simulink model "gsm_gprs_sim900_demo"  (Simulink 7.3)
settings: Solver=FixedStepDiscrete  SolverMode=SingleTasking  StartTime=0.0  StopTime=10.0  RelTol=1e-3
PreLoadFcn:
  | waijung.modelPreload; % Required for working with Waijung Blockset. Do not remove.
undefined symbols (not defined in the file): HSEOSC, Link, LQFP176, ST, STM32F417IG
libraries: waijung_atcmd_gsmgprs_lib x4, waijung_string_manipulate x4, simulink x3, waijung_systimer_lib x2, stm32f4_device_config_lib x1, stm32f4_io_lib x1
CloseFcn:
  | waijung.modelClose; % Required for working with Waijung Blockset. Do not remove.
settings Model: Creator=Krisada  LastModifiedBy=Krisada
settings OptimizationCC: OptimizeModelRefInitCode=on  LifeSpan=1
settings HardwareCC: ProdEndianess=LittleEndian  ProdHWDeviceType=ARM Compatible->Cortex - M4  TargetEndianess=LittleEndian  TargetHWDeviceType=ARM Compatible->Cortex - M4
settings RTWCC: SystemTargetFile=stm32f4.tlc  GenerateMakefile=off  TemplateMakefile=ert_default_tmf  Description=STM32F4 Target  ProcessScript=stm32f4_make_rtw_hook
settings CodeAppCC: IgnoreCustomStorageClasses=off
settings STFCustomTargetCC: ModelReferenceCompliant=off  CombineOutputUpdateFcns=on  ERTCustomFileBanners=on  SupportContinuousTime=off  SupportNonInlinedSFcns=off  SystemTargetFile=stm32f4.tlc
settings ERTTargetCC: MultiwordLength=2048  ModelReferenceCompliant=off  ParMdlRefBuildCompliant=off  CompOptLevelCompliant=off  ERTFirstTimeCompliant=off  ModelStepFunctionPrototypeControlCompliant=off  CPPClassGenCompliant=off  ExtModeMexFile=noextcomm  InlinedParameterPlacement=NonHierarchical  ERTSrcFileBannerTemplate=stm32f4_code_template.cgt  ERTHdrFileBannerTemplate=stm32f4_code_template.cgt  ERTDataSrcFileTemplate=stm32f4_code_template.cgt  ERTDataHdrFileTemplate=stm32f4_code_template.cgt  ERTCustomFileTemplate=stm32f4_file_process.tlc

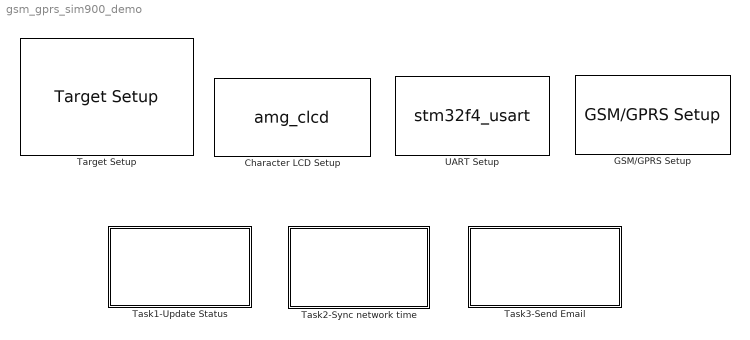
== system gsm_gprs_sim900_demo ==
  Character LCD Setup : S-Function  FunctionName=amg_clcd  Parameters=module,configuration,inputtypearray,outputtypearray,confstr,sampletime,sampletimestr,blockid  EnableBusSupport=off  mask(amg_clcd){configuration=Setup, module=1, model=amg CLCD Std, interface=4-bits, linecount=4, columncount=16, gpiotype=Push-pull, controlport=E, control_rs=7, control_rw=8, control_en=9, dataport=E, data0=12, data1=13, data2=14, data3=15, usestringbuffer=off, stringbuffer=<empty>, varname=, inputtypearray=[0], outputtypearray=[0], confstr=["4","4","16","PP","E","7","9","8","","E","","","","","12","13","14","15","0","","0","0","0","0","1","0","0","0","0","stm32f4"], sampletime=-1, sampletimestr=0.01, blockid=CharacterLCDSetup}
      mask prompts: model "LCD model:"; linecount "Number of lines (2 or 4):"; columncount "Number of columns (16 or 20):"; gpiotype "GPIO Output type:"; controlport "GPIO control port:"; control_rs "GPIO control pin, RS:"; control_rw "GPIO control pin, RW:"; control_en "GPIO control pin, EN:"; dataport "GPIO data D[7:4] port"; data0 "GPIO data pin, D4:"; data1 "GPIO data pin, D5:"; data2 "GPIO data pin, D6:"; data3 "GPIO data pin, D7:"; usestringbuffer "Use string buffer"; stringbuffer "String buffer"; varname "Variable name"; inputtypearray "Input type array"; outputtypearray "Output type array"; confstr "Configuration string"; sampletime "Sample time (sec)"; sampletimestr "Compiled sample time (sec) in string"
      mask init:
      | amg_clcd_callback('init');
      mask Help: web(fullfile(waijungdocroot,'amg_clcd_setup.htm'), '-browser')
      mask StyleString: popup(Setup|Transaction),popup(1|2|3|4),popup(amg CLCD Std),popup(4-bits),edit,edit,popup(Push-pull|Open-drain),popup(A|B|C|D|E|F|G|H|I),popup(0|1|2|3|4|5|6|7|8|9|10|11|12|13|14|15),popup(0|1|2|3|4|5|6|7|8|9|10|11|12|13|14|15),popup(0|1|2|3|4|5|6|7|8|9|10|11|12|13|14|15),popup(A|B|C|D|E|F|G|H|I),popup(0|1|2|3|4|5|6|7|8|9|10|11|12|13|14|15),popup(0|1|2|3|4|5|6|7|8|9|10|11|12|13|14|15),popup(0|1|2|3|4|5|6|7|8|9|10|11|12|13|14|15),popup(0|1|2|3|4|5|6|7|8|9|10|11|12|13|14|15),checkbox,popup(<empty>),edit,edit,edit,edit,edit,edit,edit
      mask CallbackString: amg_clcd_callback('configuration');||||||||||||||||amg_clcd_callback('usestringbuffer');||amg_clcd_callback('varname');|||amg_clcd_callback('confstr');|amg_clcd_callback('sampletime');|amg_clcd_callback('sampletimestr');|amg_clcd_callback('blockid');
      mask Display: text(0.5, 0.5, 'Module: CLCD1 (Setup)\nInterface: 4-bits\nCntrl: E7/E8/E9\nD[7:4]: E12/E13/E14/E15\nTs (sec): 0.01','ver','middle','hor','center');
  GSM/GPRS Setup : waijung_atcmd_gsmgprs_lib/GSM//GPRS Setup  conf=Setup  uartmodule=2  connectiontype=GPRS  apn='Internet'  user=''  password=''  pwrkey_port=D  pwrkey_pin=1  reset_port=D  reset_pin=0  portpinstr=0  sampletime=inf  blockid=GSMGPRSSetup  inputporttype=[]  inputportwidth=[]  inputportlabel={}  outputporttype=[]  outputportwidth=[]  outputportlabel={}  compat=0  optionstring="[\"1\",\"2\",\"GPRS\",\"Internet\",\"D\",\"1\",\"D\",\"0\",\"0\",\"\",\"''\",\"''\"]"  stringparam1=''  stringparam2=''  stringparam3=''  stringparam4=''
  Target Setup : stm32f4_device_config_lib/Target Setup  Priority=100  compiler=GNU ARM  previous_compiler=GNU ARM  mcu=STM32F417IG (LQFP176)  mcustr=STM32F417IG  clockconfig=HSEOSC-8MHz  system_stm32f4xx_c_path=F:\trunk\targets\stm32f4_target\stm32f4\utils\system_stm32f4xx_default\STM32F40_41xxx\hseosc8mhz  showmemoryconfiguration=on  stacksize=0x2000  heapsize=0x2000  enableautocompiledownload=on  fullchiperase=off  programmerinterface=ST-Link  editctrlstr=on  compilercontrolstr=$(patsubst %, -I%, .) -mcpu=cortex-m4 -mthumb -mthumb-interwork -mfloat-abi=hard -mfpu=fpv4-sp-d16 -ffast-math -Wall -Wextra -Ofast  assemblercontrolstr=$(patsubst %, -I%, .) -mcpu=cortex-m4 -mthumb -mthumb-interwork -mfloat-abi=hard -mfpu=fpv4-sp-d16 -ffast-math -Wall -Wextra -Ofast -Wa,-amhls=$(<:.s=.lst) -D__STACK_SIZE=$(STACK_SIZE) -D__HEAP_SIZE=$(HEAP_SIZE)  linkercontrolstr=-T$(LD_SCRIPT) -g -Wl,-Map=$(MAP),--cref,--no-warn-mismatch -mcpu=cortex-m4 -mthumb -mthumb-interwork -mfloat-abi=hard -mfpu=fpv4-sp-d16 -specs=nosys.specs  runafterdownload=on  execprofile=None  profileruart=3  profilerbaud=500000  profilertxpin=D8  profilerinitstr=0.01,168000000,1680000,500000,0  manualsetsampletime=on  sampletime=0.01  blockid=TargetSetup  systickreloadvalue=1680000  hseval=8000000  lastprofileruart=3  hclk=168000000  flashorigin=0x8000000  flashlength=1024k  ramorigin=0x20000000  ramlength=128k  useextram=off
  Task1-Update Status : Subsystem
  Task2-Sync network time : Subsystem
  Task3-Send Email : Subsystem
  UART Setup : S-Function  Priority=1  FunctionName=stm32f4_usart  Parameters=configuration,uartmodule,transfer,baudrate,inputtype,outputtype,confstr,binheaderarray,binterminatorarray,asciiheader,asciiterminator,bindatalength,packetmode,varname,sampletime,sampletimestr,blockid  EnableBusSupport=off  mask(stm32f4_usart){configuration=Setup, uartmodule=2, baudrate=115200, databits=8, parity=No, stopbit=1, remaptxpin=D5, remaprxpin=D6, flowcontrol=None, remapctspin=Not used, remaprtspin=Not used, advanceoptions=on, rxbuffersize=2048, txbuffersize=2048, transfer=Blocking, packetmode=Ascii, binheader='7E 7E', binterminator='03 03', porttype_double=1, porttype_single=0, porttype_int8=1, porttype_uint8=0, porttype_int16=0, porttype_uint16=0, porttype_int32=0, porttype_uint32=0, asciiformat='%d,%f', rx_asciiterminator=CRLF (0x0D 0x0A - "\r\n"), tx_asciiterminator=CR (0x0D - "\r"), storagename=<empty>, varname=, inputtype=[0], outputtype=[0], binheaderarray=[0], binterminatorarray=[0], bindatalength=0, asciiheader='', asciiterminator=[0], sampletime=-1, sampletimestr=0.01, blockid=UARTSetup, confstr=[ "dummy", "1", "D", "5", "1", "D", "6", "0", "*", "*", "0", "*", "*", "1", "4", "6", "1", "4", "5", "2048", "2048", "1", "2", "115200", "8", "No", "1", "None", "USART2"], lastmodule=2}
      mask prompts: uartmodule "UART Module"; baudrate "Baud rate (bps)"; databits "Data bits"; stopbit "Stop bit"; remaptxpin "Tx Pin"; remaprxpin "Rx Pin"; flowcontrol "Hardware flow control"; remapctspin "HW Flow control, CTS Pin"; remaprtspin "HW Flow control, RTS Pin"; advanceoptions "Advance options"; rxbuffersize "Rx buffer size (bytes)"; txbuffersize "Tx buffer size (bytes)"; packetmode "Packet mode"; binheader "Binary header (example: '7E 7E')"; binterminator "Binary terminator (example: '03 03')"; porttype_double "Number of data port, type DOUBLE"; porttype_single "Number of data port, type SINGLE"; porttype_int8 "Number of data port, type INT8"; porttype_uint8 "Number of data port, type UINT8"; porttype_int16 "Number of data port, type INT16"; porttype_uint16 "Number of data port, type UINT16"; porttype_int32 "Number of data port, type INT32"; porttype_uint32 "Number of data port, type UINT32"; asciiformat "Ascii format"; rx_asciiterminator "End of packet"; tx_asciiterminator "End of packet"; storagename "Buffer"; varname "Var name"; inputtype "Input data type"; outputtype "Output data type"; binheaderarray "Binary header"; binterminatorarray "Binary terminator"; bindatalength "Binary data length"; asciiheader "Ascii header (printf format)"; asciiterminator "Ascii terminator"; sampletime "Sample time (sec)"; sampletimestr "Compiled sample time (sec) in string"; confstr "Configuration string"; lastmodule "Last module selected"
      mask help:
      | Default STM32F4DISCOVERY + aMG F4 Connect 2 + aMG USB Converter N2 settings use
      |
      | USART3, Tx D8, Rx D9 and USB Serial Converter A.
      mask init:
      | stm32f4_usart_callback('init');
      mask Help: web(fullfile(waijungdocroot,'stm32f4_usart_setup.htm'), '-browser')
      mask StyleString: popup(Setup|Tx|Rx),popup(1|2|3|4|5|6),edit,popup(8),popup(No|Odd|Even),popup(0.5|1|1.5|2),popup(Not used|A2|D5),popup(Not used|A3|D6),popup(None|RTS|CTS|RTS/CTS),popup(Not used|A0|D3),popup(Not used|A1|D4),checkbox,popup(16|32|64|128|256|512|1024|2048),popup(16|32|64|128|256|512|1024|2048),popup(Blocking|Non-Blocking),popup(Ascii|Binary|String Buffer),edit,edit,edit,edit,edit,edit,edit,edit,edit,edit,edit,popup(CR (0x0D - "\r")|LF (0x0A - "\n")|CRLF (0x0D 0x0A - "\r\n")),popup(CR (0x0D - "\r")|LF (0x0A - "\n")|CRLF (0x0D 0x0A - "\r\n")|None),popup(<empty>),edit,edit,edit,edit,edit,edit,edit,edit,edit,edit,edit,edit,edit
      mask CallbackString: stm32f4_usart_callback('configuration');|stm32f4_usart_callback('uartmodule');|stm32f4_usart_callback('baudrate');||||||stm32f4_usart_callback('flowcontrol');|||stm32f4_usart_callback('advanceoptions');|||stm32f4_usart_callback('transfer');|stm32f4_usart_callback('packetmode');|stm32f4_usart_callback('binheader');|stm32f4_usart_callback('binterminator');|stm32f4_usart_callback('porttype');|stm32f4_usart_callback('porttype');|stm32f4_usart_callback('porttype');|stm32f4_usart_callback('porttype');|stm32f4_usart_callback('porttype');|stm32f4_usart_callback('porttype');|stm32f4_usart_callback('porttype');|stm32f4_usart_callback('porttype');|stm32f4_usart_callback('asciiformat');|stm32f4_usart_callback('rx_asciiterminator');|stm32f4_usart_callback('tx_asciiterminator');|stm32f4_usart_callback('storagename');|stm32f4_usart_callback('varname');||||||||stm32f4_usart_callback('sampletime');|stm32f4_usart_callback('sampletimestr');|stm32f4_usart_callback('blockid');||
      mask Display: text(0.5, 0.5, 'Module: USART2_Setup\nBaud (Bps): 115200\nDMA Buffer: 2048/2048\nTx/Rx Pin: D5/D6','ver','middle','hor','center');

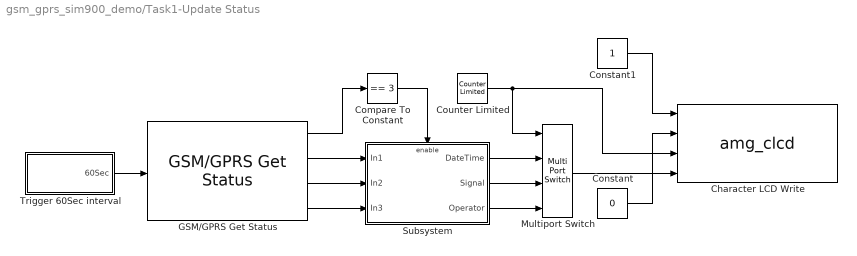
== system gsm_gprs_sim900_demo/Task1-Update Status ==
  Character LCD Write : S-Function  FunctionName=amg_clcd  Parameters=module,configuration,inputtypearray,outputtypearray,confstr,sampletime,sampletimestr,blockid  EnableBusSupport=off  mask(amg_clcd){configuration=Transaction, module=1, model=amg CLCD Std, interface=4-bits, linecount=4, columncount=20, gpiotype=Push-pull, controlport=E, control_rs=15, control_rw=13, control_en=11, dataport=A, data0=7, data1=5, data2=3, data3=1, usestringbuffer=off, stringbuffer=<empty>, varname=, inputtypearray=[4 -1 -1 -1 -1], outputtypearray=[0], confstr=["4","4","20","PP","E","15","11","13","","A","","","","","7","5","3","1","0","","1","0","0","0","1","0","0","0","0","stm32f4"], sampletime=-1, sampletimestr=0.01, blockid=Task1UpdateStatusCharacterLCDWrite}
      mask prompts: model "LCD model:"; linecount "Number of lines:"; columncount "Number of columns:"; gpiotype "GPIO Output type:"; controlport "GPIO control port:"; control_rs "GPIO control pin, RS:"; control_rw "GPIO control pin, RW:"; control_en "GPIO control pin, EN:"; dataport "GPIO data D[7:4] port"; data0 "GPIO data pin, D4:"; data1 "GPIO data pin, D5:"; data2 "GPIO data pin, D6:"; data3 "GPIO data pin, D7:"; usestringbuffer "Use string buffer"; stringbuffer "String buffer"; varname "Variable name"; inputtypearray "Input type array"; outputtypearray "Output type array"; confstr "Configuration string"; sampletime "Sample time (sec)"; sampletimestr "Compiled sample time (sec) in string"
      mask help:
      | Note for cmd:
      | 1 - Clear specified LCD line display before write data to LCD.
      | Otherwise (e.g. 0) - Write data without clearing LCD Line.
      |
      | Position:
      | x = 0, First Character (from left to right)
      | y = 0, Top Line
      mask init:
      | amg_clcd_callback('init');
      mask Help: web(fullfile(waijungdocroot,'amg_clcd_write.htm'), '-browser')
      mask StyleString: popup(Setup|Transaction),popup(1|2|3|4),popup(amg CLCD Std),popup(4-bits),edit,edit,popup(Push-pull|Open-drain),popup(A|B|C|D|E|F|G|H|I),popup(0|1|2|3|4|5|6|7|8|9|10|11|12|13|14|15),popup(0|1|2|3|4|5|6|7|8|9|10|11|12|13|14|15),popup(0|1|2|3|4|5|6|7|8|9|10|11|12|13|14|15),popup(A|B|C|D|E|F|G|H|I),popup(0|1|2|3|4|5|6|7|8|9|10|11|12|13|14|15),popup(0|1|2|3|4|5|6|7|8|9|10|11|12|13|14|15),popup(0|1|2|3|4|5|6|7|8|9|10|11|12|13|14|15),popup(0|1|2|3|4|5|6|7|8|9|10|11|12|13|14|15),checkbox,popup(<empty>),edit,edit,edit,edit,edit,edit,edit
      mask CallbackString: amg_clcd_callback('configuration');||||||||||||||||amg_clcd_callback('usestringbuffer');||amg_clcd_callback('varname');|||amg_clcd_callback('confstr');|amg_clcd_callback('sampletime');|amg_clcd_callback('sampletimestr');|amg_clcd_callback('blockid');
      mask Display: text(0.5, 0.5, 'Module: CLCD1 (Write)\nTs (sec): 0.01','ver','middle','hor','center');port_label('input', 1,'cmd');port_label('input', 2,'xpos');port_label('input', 3,'ypos');port_label('input', 4,'str');
  Compare To Constant : simulink/Logic and Bit Operations/Compare To Constant  SystemSampleTime=-1  relop===  const=3  LogicOutDataTypeMode=uint8  ZeroCross=off
  Constant : Constant  Value=0  OutDataTypeMode=uint8  OutDataType=fixdt(1, 16)  OutScaling=2^0  OutDataTypeStr=uint8
  Constant1 : Constant  OutDataTypeMode=uint8  OutDataType=fixdt(1, 16)  OutScaling=2^0  OutDataTypeStr=uint8
  Counter Limited : simulink/Sources/Counter Limited  SystemSampleTime=-1  uplimit=2  tsamp=-1
  GSM/GPRS Get Status : waijung_atcmd_gsmgprs_lib/GSM//GPRS Get Status  conf=GetStatus  portpinstr=0  sampletime=inf  blockid=Task1UpdateStatusGSMGPRSGetStatus  inputporttype=[3]  inputportwidth=[1]  inputportlabel={'Trig'}  outputporttype=[3 7 3 7]  outputportwidth=[1 6 32 1]  outputportlabel={'Status','Date/Time','Operator','Signal Strength'}  compat=0  optionstring="[\"1\",\"2\",\"GPRS\",\"Internet\",\"D\",\"1\",\"D\",\"0\",\"0\",\"\",\"\",\"\"]"  stringparam1=''  stringparam2=''
  Multiport Switch : MultiPortSwitch  zeroidx=on  OutDataType=fixdt(1, 16)  OutScaling=2^0
  Subsystem : Subsystem
  Trigger 60Sec interval : Subsystem
  wires:
  Trigger 60Sec interval/1(60Sec) -> GSM/GPRS Get Status/1
  GSM/GPRS Get Status/2 -> Subsystem/1(In1)
  GSM/GPRS Get Status/4 -> Subsystem/3(In3)
  GSM/GPRS Get Status/3 -> Subsystem/2(In2)
  GSM/GPRS Get Status/1 -> Compare To Constant/1
  Compare To Constant/1 -> Subsystem/Enable
  Subsystem/3(Operator) -> Multiport Switch/4
  Subsystem/2(Signal) -> Multiport Switch/3
  Multiport Switch/1 -> Character LCD Write/4
  Counter Limited/1 -> Multiport Switch/1, Character LCD Write/3
  Constant/1 -> Character LCD Write/2
  Constant1/1 -> Character LCD Write/1
  Subsystem/1(DateTime) -> Multiport Switch/2

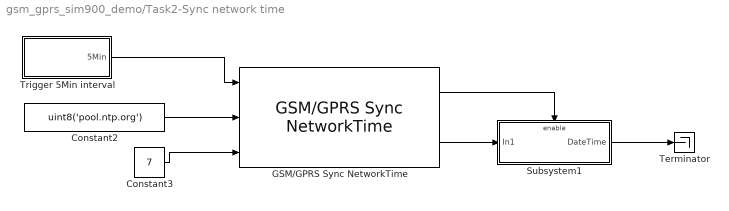
== system gsm_gprs_sim900_demo/Task2-Sync network time ==
  Constant2 : Constant  Value=uint8('pool.ntp.org')  OutDataType=fixdt(1, 16)  OutScaling=2^0
  Constant3 : Constant  Value=7  OutDataTypeMode=int32  OutDataType=fixdt(1, 16)  OutScaling=2^0  OutDataTypeStr=int32
  GSM/GPRS Sync NetworkTime : waijung_atcmd_gsmgprs_lib/GSM//GPRS Sync NetworkTime  conf=SyncNetworkTime  portpinstr=0  sampletime=inf  blockid=Task2SyncnetworktimeGSMGPRSSyncNetworkTime  inputporttype=[3 3 6]  inputportwidth=[1 -1 1]  inputportlabel={'Trig','NTP Server','Time zone'}  outputporttype=[3 7]  outputportwidth=[1 6]  outputportlabel={'Status','Date/Time'}  compat=0  optionstring="[\"1\",\"2\",\"GPRS\",\"Internet\",\"D\",\"1\",\"D\",\"0\",\"0\",\"\",\"\",\"\"]"  stringparam1=''  stringparam2=''
  Subsystem1 : Subsystem
  Terminator : Terminator
  Trigger 5Min interval : Subsystem
  wires:
  Constant2/1 -> GSM/GPRS Sync NetworkTime/2
  Constant3/1 -> GSM/GPRS Sync NetworkTime/3
  GSM/GPRS Sync NetworkTime/1 -> Subsystem1/Enable
  GSM/GPRS Sync NetworkTime/2 -> Subsystem1/1(In1)
  Trigger 5Min interval/1(5Min) -> GSM/GPRS Sync NetworkTime/1
  Subsystem1/1(DateTime) -> Terminator/1

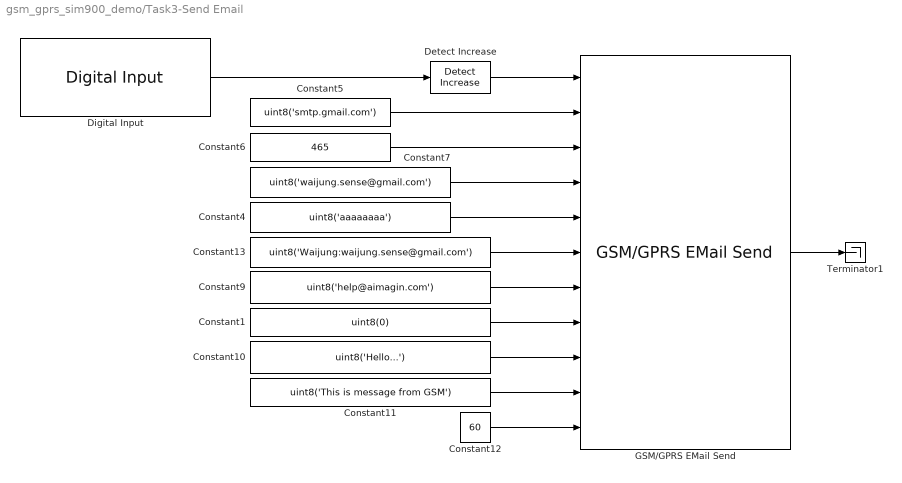
== system gsm_gprs_sim900_demo/Task3-Send Email ==
  Constant1 : Constant  Value=uint8(0)  OutDataType=fixdt(1, 16)  OutScaling=2^0
  Constant10 : Constant  Value=uint8('Hello...')  OutDataType=fixdt(1, 16)  OutScaling=2^0
  Constant11 : Constant  Value=uint8('This is message from GSM')  OutDataType=fixdt(1, 16)  OutScaling=2^0
  Constant12 : Constant  Value=60  OutDataTypeMode=int32  OutDataType=fixdt(1, 16)  OutScaling=2^0  OutDataTypeStr=int32
  Constant13 : Constant  Value=uint8('Waijung:waijung.sense@gmail.com')  OutDataType=fixdt(1, 16)  OutScaling=2^0
  Constant4 : Constant  Value=uint8('aaaaaaaa')  OutDataType=fixdt(1, 16)  OutScaling=2^0
  Constant5 : Constant  Value=uint8('smtp.gmail.com')  OutDataType=fixdt(1, 16)  OutScaling=2^0
  Constant6 : Constant  Value=465  OutDataTypeMode=uint32  OutDataType=fixdt(1, 16)  OutScaling=2^0  OutDataTypeStr=uint32
  Constant7 : Constant  Value=uint8('waijung.sense@gmail.com')  OutDataType=fixdt(1, 16)  OutScaling=2^0
  Constant9 : Constant  Value=uint8('help@aimagin.com')  OutDataType=fixdt(1, 16)  OutScaling=2^0
  Detect Increase : simulink/Logic and Bit Operations/Detect Increase  SystemSampleTime=-1  vinit=0.0
  Digital Input : stm32f4_io_lib/Digital Input  port=B  speed=100  porttype=None  porttypestr=NOPULL  use_pin0=off  use_pin1=off  use_pin2=on  use_pin3=off  use_pin4=off  use_pin5=off  use_pin6=off  use_pin7=off  use_pin8=off  use_pin9=off  use_pin10=off  use_pin11=off  use_pin12=off  use_pin13=off  use_pin14=off  use_pin15=off  pinstr=GPIO_Pin_2  usedpinarray="[0  0  1  0  0  0  0  0  0  0  0  0  0  0  0  0]"  bitbandingstr="#define Task3SendEmailDigitalInput_B2 Peripheral_BB(GPIOB->IDR, 2)  /* Output pin */"  sampletime=0.01  sampletimestr=0.01  blockid=Task3SendEmailDigitalInput  enablecustomportlabel=off  glabalinit=off  cinputportlabel=In1, In2  coutputportlabel=Out1, Out2
  GSM/GPRS EMail Send : waijung_atcmd_gsmgprs_lib/GSM//GPRS EMail Send  conf=SMTP  ssl=on  portpinstr=0  sampletime=inf  blockid=Task3SendEmailGSMGPRSEMailSend  inputporttype=[3 3 -1 3 3 3 3 3 3 3 -1]  inputportwidth=[1 -1 1 -1 -1 -1 -1 -1 -1 -1 1]  inputportlabel={'Trig','ServerName','ServerPort','***Login User','***Login Password','Sender','To Recipient','Cc Recipient','Subject','Message','Timeout(sec)'}  outputporttype=[3]  outputportwidth=[1]  outputportlabel={'Status'}  compat=0  optionstring="[\"1\",\"2\",\"GPRS\",\"Internet\",\"D\",\"1\",\"D\",\"0\",\"1\",\"\",\"\",\"\"]"  stringparam1=''  stringparam2=''
  Terminator1 : Terminator
  wires:
  Constant5/1 -> GSM/GPRS EMail Send/2
  Constant12/1 -> GSM/GPRS EMail Send/11
  Constant10/1 -> GSM/GPRS EMail Send/9
  Constant6/1 -> GSM/GPRS EMail Send/3
  Detect Increase/1 -> GSM/GPRS EMail Send/1
  Constant7/1 -> GSM/GPRS EMail Send/4
  Constant4/1 -> GSM/GPRS EMail Send/5
  Constant13/1 -> GSM/GPRS EMail Send/6
  GSM/GPRS EMail Send/1 -> Terminator1/1
  Digital Input/1 -> Detect Increase/1
  Constant9/1 -> GSM/GPRS EMail Send/7
  Constant11/1 -> GSM/GPRS EMail Send/10
  Constant1/1 -> GSM/GPRS EMail Send/8

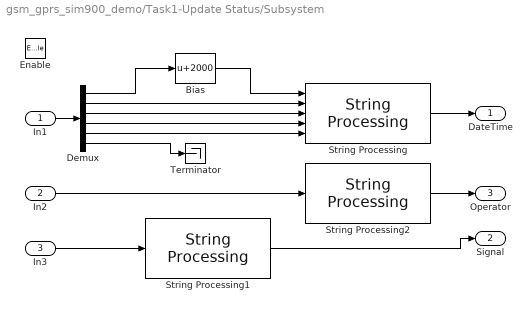
== system gsm_gprs_sim900_demo/Task1-Update Status/Subsystem ==
  In1 : Inport
  In2 : Inport  Port=2
  In3 : Inport  Port=3
  Enable : EnablePort
  Bias : Bias  Bias=2000
  Demux : Demux  Outputs=6
  String Processing : waijung_string_manipulate/String Processing  conf=processing  stringfunction=sprintf  stringformat='%u/%u/%u %u:%u'  begindelimiter=''  enddelimiter=''  buffersize=32  enablestatus=off  portpinstr=0  sampletime=inf  blockid=Task1UpdateStatusSubsystemStringProcessing  inputporttype=[-1 -1 -1 -1 -1]  inputportwidth=[1 1 1 1 1]  inputportlabel={'%u','%u','%u','%u','%u'}  outputporttype=[3]  outputportwidth=[32]  outputportlabel={'Output'}  compat=0  optionstring=[]  datatypestring="[\"uint32_t\",\"uint32_t\",\"uint32_t\",\"uint32_t\",\"uint32_t\"]"
  String Processing1 : waijung_string_manipulate/String Processing  conf=processing  stringfunction=sprintf  stringformat='Signal: %d'  begindelimiter=''  enddelimiter=''  buffersize=32  enablestatus=off  portpinstr=0  sampletime=inf  blockid=Task1UpdateStatusSubsystemStringProcessing1  inputporttype=[-1]  inputportwidth=[1]  inputportlabel={'%d'}  outputporttype=[3]  outputportwidth=[32]  outputportlabel={'Output'}  compat=0  optionstring=[]  datatypestring="[\"int32_t\"]"
  String Processing2 : waijung_string_manipulate/String Processing  conf=processing  stringfunction=sprintf  stringformat='OP: %s'  begindelimiter=''  enddelimiter=''  buffersize=32  enablestatus=off  portpinstr=0  sampletime=inf  blockid=Task1UpdateStatusSubsystemStringProcessing2  inputporttype=[3]  inputportwidth=[-1]  inputportlabel={'%s'}  outputporttype=[3]  outputportwidth=[32]  outputportlabel={'Output'}  compat=0  optionstring=[]  datatypestring="[\"char *\"]"
  Terminator : Terminator
  DateTime : Outport  InitialOutput="uint8('Search network..                ')"
  Signal : Outport  Port=2  InitialOutput="uint8('                                ')"
  Operator : Outport  Port=3  InitialOutput="uint8('                                ')"
  wires:
  Demux/1 -> Bias/1
  Demux/2 -> String Processing/2
  Demux/3 -> String Processing/3
  Demux/4 -> String Processing/4
  Demux/5 -> String Processing/5
  In1/1 -> Demux/1
  String Processing/1 -> DateTime/1
  In3/1 -> String Processing1/1
  String Processing1/1 -> Signal/1
  In2/1 -> String Processing2/1
  Bias/1 -> String Processing/1
  Demux/6 -> Terminator/1
  String Processing2/1 -> Operator/1

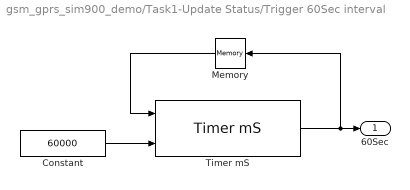
== system gsm_gprs_sim900_demo/Task1-Update Status/Trigger 60Sec interval ==
  Constant : Constant  Value=60000  OutDataTypeMode=uint32  OutDataType=fixdt(1, 16)  OutScaling=2^0  OutDataTypeStr=uint32
  Memory : Memory  InheritSampleTime=on  LinearizeMemory=on  LinearizeAsDelay=on
  Timer mS : waijung_systimer_lib/Timer mS  conf=timerms  mode=Non-blocking  portpinstr=0  sampletime=inf  blockid=Task1UpdateStatusTrigger60SecintervalTimermS  inputporttype=[3 7]  inputportwidth=[]  inputportlabel={'Reset','mS'}  outputporttype=[3]  outputportwidth=[]  outputportlabel={'Timeout'}  compat=0  optionstring="[\"Non-blocking\"]"
  60Sec : Outport
  wires:
  Timer mS/1 -> Memory/1, 60Sec/1
  Memory/1 -> Timer mS/1
  Constant/1 -> Timer mS/2

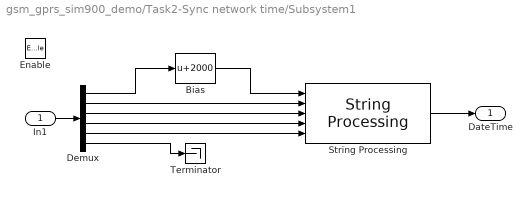
== system gsm_gprs_sim900_demo/Task2-Sync network time/Subsystem1 ==
  In1 : Inport
  Enable : EnablePort
  Bias : Bias  Bias=2000
  Demux : Demux  Outputs=6
  String Processing : waijung_string_manipulate/String Processing  conf=processing  stringfunction=sprintf  stringformat='%u/%u/%u %u:%u'  begindelimiter=''  enddelimiter=''  buffersize=32  enablestatus=off  portpinstr=0  sampletime=inf  blockid=Task2SyncnetworktimeSubsystem1StringProcessing  inputporttype=[-1 -1 -1 -1 -1]  inputportwidth=[1 1 1 1 1]  inputportlabel={'%u','%u','%u','%u','%u'}  outputporttype=[3]  outputportwidth=[32]  outputportlabel={'Output'}  compat=0  optionstring=[]  datatypestring="[\"uint32_t\",\"uint32_t\",\"uint32_t\",\"uint32_t\",\"uint32_t\"]"
  Terminator : Terminator
  DateTime : Outport
  wires:
  Demux/6 -> Terminator/1
  Bias/1 -> String Processing/1
  String Processing/1 -> DateTime/1
  In1/1 -> Demux/1
  Demux/5 -> String Processing/5
  Demux/4 -> String Processing/4
  Demux/3 -> String Processing/3
  Demux/2 -> String Processing/2
  Demux/1 -> Bias/1

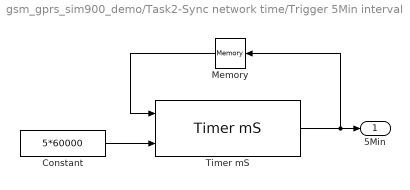
== system gsm_gprs_sim900_demo/Task2-Sync network time/Trigger 5Min interval ==
  Constant : Constant  Value=5*60000  OutDataTypeMode=uint32  OutDataType=fixdt(1, 16)  OutScaling=2^0  OutDataTypeStr=uint32
  Memory : Memory  InheritSampleTime=on  LinearizeMemory=on  LinearizeAsDelay=on
  Timer mS : waijung_systimer_lib/Timer mS  conf=timerms  mode=Non-blocking  portpinstr=0  sampletime=inf  blockid=Task2SyncnetworktimeTrigger5MinintervalTimermS  inputporttype=[3 7]  inputportwidth=[]  inputportlabel={'Reset','mS'}  outputporttype=[3]  outputportwidth=[]  outputportlabel={'Timeout'}  compat=0  optionstring="[\"Non-blocking\"]"
  5Min : Outport
  wires:
  Constant/1 -> Timer mS/2
  Memory/1 -> Timer mS/1
  Timer mS/1 -> 5Min/1, Memory/1
